simulink model "steps"  (R2018a)
settings: Solver=VariableStepAuto  StartTime=0.0  StopTime=ttotal  RelTol=1e-3
settings Model: Creator=Carlos  LastModifiedBy=Carlos

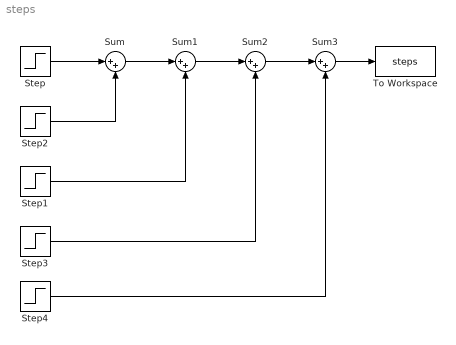
== system steps ==
  Step : Step  SampleTime=0
  Step1 : Step  Time=10  After=2  SampleTime=0
  Step2 : Step  Time=6  After=-1  SampleTime=0
  Step3 : Step  Time=14  After=-1  SampleTime=0
  Step4 : Step  Time=18  SampleTime=0
  Sum{,1..3} (4 alike) : Sum  Inputs=|++
  To Workspace : ToWorkspace  VariableName=steps  SampleTime=-1
  wires:
  Sum3/1 -> To Workspace/1
  Sum2/1 -> Sum3/1
  Sum1/1 -> Sum2/1
  Sum/1 -> Sum1/1
  Step/1 -> Sum/1
  Step2/1 -> Sum/2
  Step1/1 -> Sum1/2
  Step3/1 -> Sum2/2
  Step4/1 -> Sum3/2
